simulink model "project1_week3"  (R2020b)
settings: Solver=VariableStepAuto  StartTime=0.0  StopTime=10.0  RelTol=1e-3
settings Model: Creator=RASIKA MALGI  LastModifiedBy=RASIKA MALGI

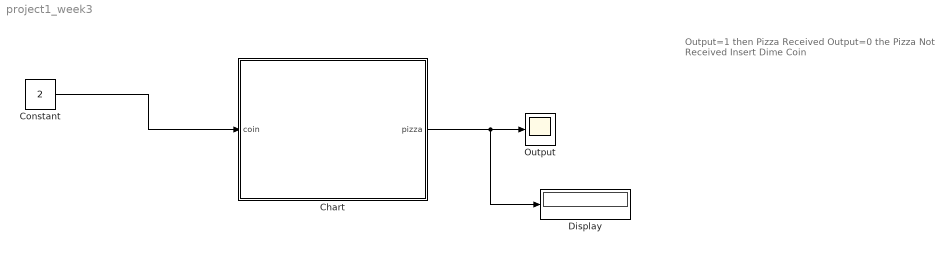
== system project1_week3 ==
  note: Output=1 then Pizza Received
      | Output=0 the Pizza Not Received Insert Dime Coin
  Chart : Stateflow chart  TreatAsAtomicUnit=on
  Constant : Constant  Value=2
  Display : Display
  Output : Scope
  wires:
  Constant/1 -> Chart/1(coin)
  Chart/1(pizza) -> Display/1, Output/1

== stateflow chart project1_week3/Chart ==
  state Nickel
  state Zero
  state Dime
  (default) -> Zero
  Zero -> Nickel [order 1] : [coin==1]{pizza=0}
  Nickel -> Zero [order 2] : [coin==2]{pizza==1}
  Nickel -> Dime [order 1] : [coin==1]{pizza=0}
  Dime -> Nickel [order 2] : [coin==0]{pizza=1}
  Dime -> Zero [order 1] : [coin==1]{pizza=1}
  Zero -> Dime [order 2] : [coin==2]{pizza=0}
  data: coin input; pizza output
